simulink model "VAS_LEVEL0_TASK0_MAIN"  (Simulink 3.00)

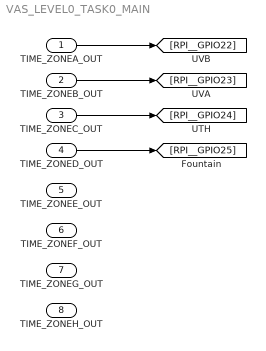
== system VAS_LEVEL0_TASK0_MAIN ==
  TIME_ZONEA_OUT : Inport  Port=1
  TIME_ZONEB_OUT : Inport  Port=2
  TIME_ZONEC_OUT : Inport  Port=3
  TIME_ZONED_OUT : Inport  Port=4
  TIME_ZONEE_OUT : Inport  Port=5
  TIME_ZONEF_OUT : Inport  Port=6
  TIME_ZONEG_OUT : Inport  Port=7
  TIME_ZONEH_OUT : Inport  Port=8
  wires:
  TIME_ZONEA_OUT/1 -> [RPI__GPIO22]
  TIME_ZONEB_OUT/1 -> [RPI__GPIO23]
  TIME_ZONEC_OUT/1 -> [RPI__GPIO24]
  TIME_ZONED_OUT/1 -> [RPI__GPIO25]
